simulink model "sum_complex_test"  (Simulink 8.4)
settings: Solver=VariableStepDiscrete  StartTime=0.0  StopTime=10.0  RelTol=1e-3
settings Model: Creator=arnaud  LastModifiedBy=arnaud
settings DataIOCC: SaveFormat=Structure

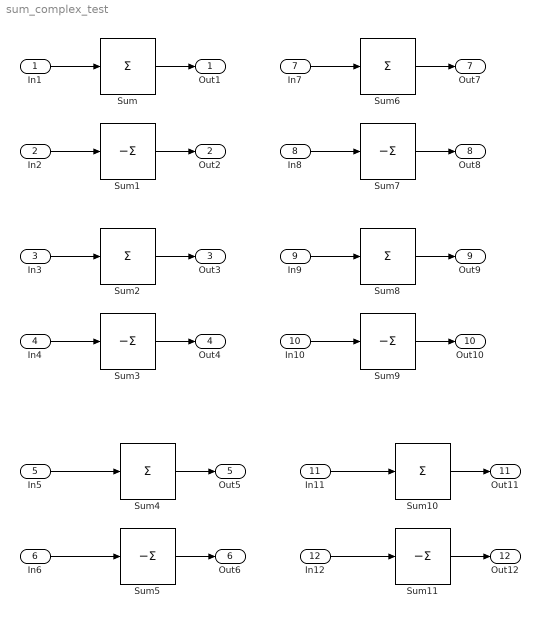
== system sum_complex_test ==
  In1 : Inport
      settings: SignalType=complex
  In2 : Inport  Port=2
      settings: SignalType=complex
  In3 : Inport  Port=3  PortDimensions=3
      settings: SignalType=complex
  In4 : Inport  Port=4  PortDimensions=3
      settings: SignalType=complex
  In5 : Inport  Port=5  PortDimensions=[2 3]
      settings: SignalType=complex
  In6 : Inport  Port=6  PortDimensions=[2 3]
      settings: SignalType=complex
  In7 : Inport  Port=7  OutDataTypeStr=int8
      settings: SignalType=complex
  In8 : Inport  Port=8  OutDataTypeStr=int8
      settings: SignalType=complex
  In9 : Inport  Port=9  OutDataTypeStr=int8  PortDimensions=3
      settings: SignalType=complex
  In10 : Inport  Port=10  OutDataTypeStr=int8  PortDimensions=3
      settings: SignalType=complex
  In11 : Inport  Port=11  OutDataTypeStr=int8  PortDimensions=[2 3]
      settings: SignalType=complex
  In12 : Inport  Port=12  OutDataTypeStr=int8  PortDimensions=[2 3]
      settings: SignalType=complex
  Sum{,2,4,6,8,10} (6 alike) : Sum  Inputs=+
  Sum{1,3,5,7,9,11} (6 alike) : Sum  Inputs=-
  Out1 : Outport
  Out2 : Outport  Port=2
  Out3 : Outport  Port=3
  Out4 : Outport  Port=4
  Out5 : Outport  Port=5
  Out6 : Outport  Port=6
  Out7 : Outport  Port=7
  Out8 : Outport  Port=8
  Out9 : Outport  Port=9
  Out10 : Outport  Port=10
  Out11 : Outport  Port=11
  Out12 : Outport  Port=12
  wires:
  In1/1 -> Sum/1
  Sum/1 -> Out1/1
  In7/1 -> Sum6/1
  Sum6/1 -> Out7/1
  In2/1 -> Sum1/1
  Sum1/1 -> Out2/1
  In3/1 -> Sum2/1
  Sum2/1 -> Out3/1
  In4/1 -> Sum3/1
  Sum3/1 -> Out4/1
  In5/1 -> Sum4/1
  Sum4/1 -> Out5/1
  In6/1 -> Sum5/1
  Sum5/1 -> Out6/1
  In8/1 -> Sum7/1
  Sum7/1 -> Out8/1
  In9/1 -> Sum8/1
  Sum8/1 -> Out9/1
  In10/1 -> Sum9/1
  Sum9/1 -> Out10/1
  In11/1 -> Sum10/1
  Sum10/1 -> Out11/1
  In12/1 -> Sum11/1
  Sum11/1 -> Out12/1
